simulink model "Linear_model"  (R2020b)
settings: Solver=VariableStepAuto  StartTime=0.0  StopTime=10  MaxStep=1e-6  RelTol=1e-4
values from neighbouring files (symbols this model uses):
  SS_SG = connect(rl_ss,isnb_ss,snb_ss,sg,vsg_pu,vsg,exf,exc_ss,gov_ss,turb_ss,isg_pu,wsg_pu,ang,dang,vgx_g,igx_g,input_vars,output_vars)    [SS_model.m]    (also in SS_model_pu.m = connect(tr_ss,isnb_ss,snb_ss,sg,vsg_pu,vsg,exf,exc_ss,gov_ss)
  Vb = 22e3    (= 22000)    [SG_param.m]    (also in sg_slack_POD.m = Vb_kV*1e3)
settings Model: Creator=Collados  LastModifiedBy=Collados

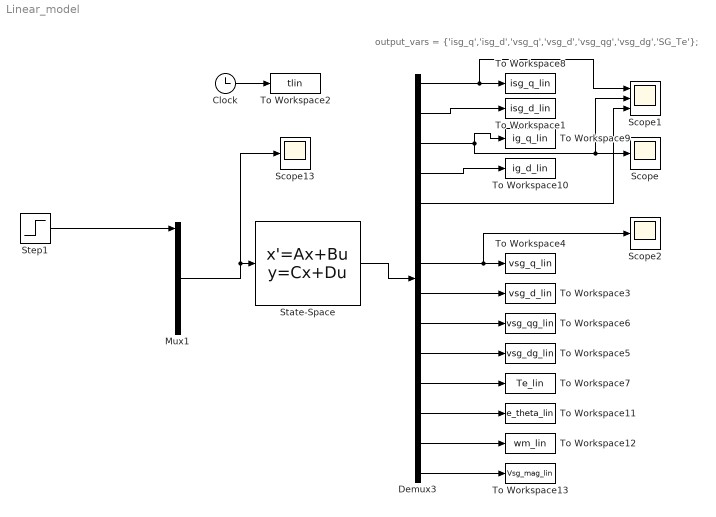
== system Linear_model ==
  note: output_vars = {'isg_q','isg_d','vsg_q','vsg_d','vsg_qg','vsg_dg','SG_Te'};
  Clock : Clock
  Demux3 : Demux  Outputs=14
  Mux1 : Mux  Inputs=length(SS_SG.InputName)
  Scope : Scope
  Scope1 : Scope  NumInputPorts=3
  Scope13 : Scope
  Scope2 : Scope
  State-Space : StateSpace  A=SS_SG.A  B=SS_SG.B  C=SS_SG.C  D=SS_SG.D  InitialCondition=zeros(length(SS_SG.A),1)
  Step1 : Step  After=Vb*sqrt(2/3)*0.005  SampleTime=0
  To Workspace1 : ToWorkspace  VariableName=isg_d_lin  SampleTime=-1
      settings: Decimation=20  Save2DSignal=2-D array (concatenate along first dimension)
  To Workspace10 : ToWorkspace  VariableName=ig_d_lin  SampleTime=-1
      settings: Decimation=20  Save2DSignal=2-D array (concatenate along first dimension)
  To Workspace11 : ToWorkspace  VariableName=e_theta_lin  SampleTime=-1
      settings: Decimation=20  Save2DSignal=2-D array (concatenate along first dimension)
  To Workspace12 : ToWorkspace  VariableName=wm_lin  SampleTime=-1
      settings: Decimation=20  Save2DSignal=2-D array (concatenate along first dimension)
  To Workspace13 : ToWorkspace  VariableName=Vsg_mag_lin  SampleTime=-1
      settings: Decimation=20  Save2DSignal=2-D array (concatenate along first dimension)
  To Workspace2 : ToWorkspace  VariableName=tlin  SampleTime=-1
      settings: Decimation=20  Save2DSignal=2-D array (concatenate along first dimension)
  To Workspace3 : ToWorkspace  VariableName=vsg_d_lin  SampleTime=-1
      settings: Decimation=20  Save2DSignal=2-D array (concatenate along first dimension)
  To Workspace4 : ToWorkspace  VariableName=vsg_q_lin  SampleTime=-1
      settings: Decimation=20  Save2DSignal=2-D array (concatenate along first dimension)
  To Workspace5 : ToWorkspace  VariableName=vsg_dg_lin  SampleTime=-1
      settings: Decimation=20  Save2DSignal=2-D array (concatenate along first dimension)
  To Workspace6 : ToWorkspace  VariableName=vsg_qg_lin  SampleTime=-1
      settings: Decimation=20  Save2DSignal=2-D array (concatenate along first dimension)
  To Workspace7 : ToWorkspace  VariableName=Te_lin  SampleTime=-1
      settings: Decimation=20  Save2DSignal=2-D array (concatenate along first dimension)
  To Workspace8 : ToWorkspace  VariableName=isg_q_lin  SampleTime=-1
      settings: Decimation=20  Save2DSignal=2-D array (concatenate along first dimension)
  To Workspace9 : ToWorkspace  VariableName=ig_q_lin  SampleTime=-1
      settings: Decimation=20  Save2DSignal=2-D array (concatenate along first dimension)
  wires:
  Mux1/1 -> Scope13/1, State-Space/1
  State-Space/1 -> Demux3/1
  Step1/1 -> Mux1/1
  Clock/1 -> To Workspace2/1
  Demux3/1 -> Scope1/1, To Workspace8/1
  Demux3/2 -> To Workspace1/1
  Demux3/3 -> Scope1/2, Scope/1, To Workspace9/1
  Demux3/4 -> To Workspace10/1
  Demux3/7 -> Scope2/1, To Workspace4/1
  Demux3/8 -> To Workspace3/1
  Demux3/9 -> To Workspace6/1
  Demux3/10 -> To Workspace5/1
  Demux3/11 -> To Workspace7/1
  Demux3/5 -> Scope1/3
  Demux3/12 -> To Workspace11/1
  Demux3/13 -> To Workspace12/1
  Demux3/14 -> To Workspace13/1
